simulink model "LEDsnake_EMO_R8_task"  (Simulink 3.00)
libraries: logiclib x7, genlib x6, mathlib x4, analoglib x2, execlib x1, inoutlib x1

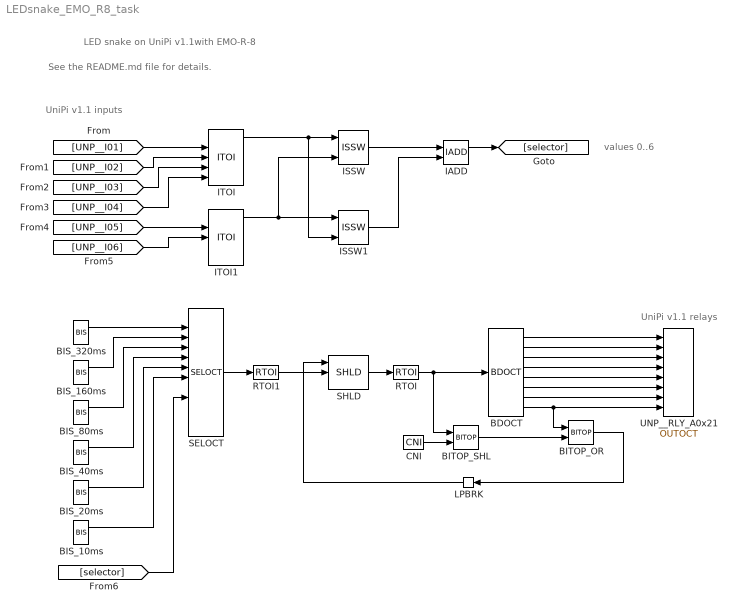
== system LEDsnake_EMO_R8_task ==
  note: UniPi v1.1 relays
  note: See the README.md file for details.
  note: UniPi v1.1 inputs
  note: values 0..6
  note: LED snake on UniPi v1.1with EMO-R-8
  BDOCT : logiclib/BDOCT  shift=0
  BIS_10ms : genlib/BIS  Y0=off  t1=0.005  t2=0.01  t3=0  t4=4  t5=5  t6=6  t7=7  t8=8  RPT=on
  BIS_160ms : genlib/BIS  Y0=off  t1=0.080  t2=0.160  t3=0  t4=4  t5=5  t6=6  t7=7  t8=8  RPT=on
  BIS_20ms : genlib/BIS  Y0=off  t1=0.01  t2=0.02  t3=0  t4=4  t5=5  t6=6  t7=7  t8=8  RPT=on
  BIS_320ms : genlib/BIS  Y0=off  t1=0.160  t2=0.320  t3=0  t4=4  t5=5  t6=6  t7=7  t8=8  RPT=on
  BIS_40ms : genlib/BIS  Y0=off  t1=0.02  t2=0.04  t3=0  t4=4  t5=5  t6=6  t7=7  t8=8  RPT=on
  BIS_80ms : genlib/BIS  Y0=off  t1=0.04  t2=0.08  t3=0  t4=4  t5=5  t6=6  t7=7  t8=8  RPT=on
  BITOP_OR : logiclib/BITOP  iop=2: Bit OR
  BITOP_SHL : logiclib/BITOP  iop=5: Shift Left
  CNI : mathlib/CNI  icn=1
  IADD : mathlib/IADD  vtype=4: Long  SAT=off
  ISSW : logiclib/ISSW
  ISSW1 : logiclib/ISSW
  ITOI : logiclib/ITOI  BINF=on  fktab=[0 1 2 0 3 0 0 0 4 0 0 0 0 0 0 0]
  ITOI1 : logiclib/ITOI  BINF=on  fktab=[0 5 6 0 0 0 0 0 0 0 0 0 0 0 0 0]
  LPBRK : execlib/LPBRK  Orientation=left
  RTOI : mathlib/RTOI
  RTOI1 : mathlib/RTOI
  SELOCT : analoglib/SELOCT  BINF=off
  SHLD : analoglib/SHLD  y0=7  mode=1: Triggered sampling
  UNP__RLY_A0x21 : inoutlib/OUTOCT
  wires:
  BDOCT/1 -> UNP__RLY_A0x21/1
  BDOCT/2 -> UNP__RLY_A0x21/2
  BDOCT/3 -> UNP__RLY_A0x21/3
  BDOCT/4 -> UNP__RLY_A0x21/4
  BDOCT/5 -> UNP__RLY_A0x21/5
  BDOCT/6 -> UNP__RLY_A0x21/6
  BDOCT/7 -> UNP__RLY_A0x21/7
  BDOCT/8 -> BITOP_OR/1, UNP__RLY_A0x21/8
  BIS_10ms/1 -> SELOCT/7
  BIS_160ms/1 -> SELOCT/3
  BIS_20ms/1 -> SELOCT/6
  BIS_320ms/1 -> SELOCT/2
  BIS_40ms/1 -> SELOCT/5
  BIS_80ms/1 -> SELOCT/4
  BITOP_OR/1 -> LPBRK/1
  BITOP_SHL/1 -> BITOP_OR/2
  CNI/1 -> BITOP_SHL/2
  [UNP__I01] -> ITOI/2
  [UNP__I02] -> ITOI/3
  [UNP__I03] -> ITOI/4
  [UNP__I04] -> ITOI/5
  [UNP__I05] -> ITOI1/2
  [UNP__I06] -> ITOI1/3
  [selector] -> SELOCT/9
  IADD/1 -> [selector]
  ISSW/1 -> IADD/1
  ISSW1/1 -> IADD/2
  ITOI/1 -> ISSW/1, ISSW1/3
  ITOI1/1 -> ISSW/3, ISSW1/1
  LPBRK/1 -> SHLD/1
  RTOI/1 -> BDOCT/1, BITOP_SHL/1
  RTOI1/1 -> SHLD/2
  SELOCT/1 -> RTOI1/1
  SHLD/1 -> RTOI/1
